simulink model "ASM_FOC_Implementation"  (R2020a)
settings: Solver=ode3  StartTime=0.0  StopTime=t_end  FixedStep=dt  RelTol=1e-3  EnableMultiTasking=on
values from neighbouring files (symbols this model uses):
  L_m = 0.326    [Experiment_4_Parameter.m]
  L_r = 0.340    (= 0.34)    [Experiment_4_Parameter.m]
  L_s = 0.340    (= 0.34)    [Experiment_4_Parameter.m]
  L_sigma_r = L_r - L_m    (= 0.014)    [Experiment_4_Parameter.m]
  L_sigma_s = L_s - L_m    (= 0.014)    [Experiment_4_Parameter.m]
  p = 1    [Experiment_4_Parameter.m]
  R_r = 2.9    [Experiment_4_Parameter.m]
  R_s = 2.3    [Experiment_4_Parameter.m]
  sigma = (L_s*L_r - L_m^2)/(L_s*L_r)    (= 0.0806574394464)    [Experiment_4_Parameter.m]
  T_c = 1/4000    (= 0.00025)    [Experiment_4_Parameter.m]
  Theta_M = 0.0022    [Experiment_4_Parameter.m]
  U_dc = 560    [Experiment_4_Parameter.m]
settings Model: Creator=julien  LastModifiedBy=ge29wel
settings DataIOCC: LimitDataPoints=on  SaveFormat=Array  ReturnWorkspaceOutputs=off
settings OptimizationCC: ExpressionDepthLimit=2147483647  LifeSpan=inf
settings DebuggingCC: UnderspecifiedInitializationDetection=Classic  MergeDetectMultiDrivingBlocksExec=none  SolverPrmCheckMsg=warning  MultiTaskRateTransMsg=warning  StateNameClashWarn=warning  SFUnexpectedBacktrackingDiag=warning  SFNoUnconditionalDefaultTransitionDiag=warning  SFExecutionAtInitializationDiag=none  ArithmeticOperatorsInVariantConditions=warning
settings HardwareCC: ProdBitPerPointer=32  ProdBitPerSizeT=32  ProdBitPerPtrDiffT=32  ProdLargestAtomicFloat=None  ProdIntDivRoundTo=Undefined  ProdEndianess=Unspecified  ProdWordSize=32  ProdHWDeviceType=32-bit Generic
settings ModelReferenceCC: PropagateSignalLabelsOutOfModel=off
settings SFSimCC: SimUseLocalCustomCode=off  CustomCodeUndefinedFunction=UseInterfaceOnly
settings RTWCC: RTWUseLocalCustomCode=off
settings CodeAppCC: StateflowObjectComments=on
settings GRTTargetCC: TargetLangStandard=C89/C90 (ANSI)
settings ConfigComp: CovMetricSettings=dw  CovHtmlReporting=on  CovSaveCumulativeToWorkspaceVar=on  CovSaveSingleToWorkspaceVar=on  CovExternalEMLEnable=off  CovSFcnEnable=off
settings ConfigurationSet: Description=SimMechanics 2G

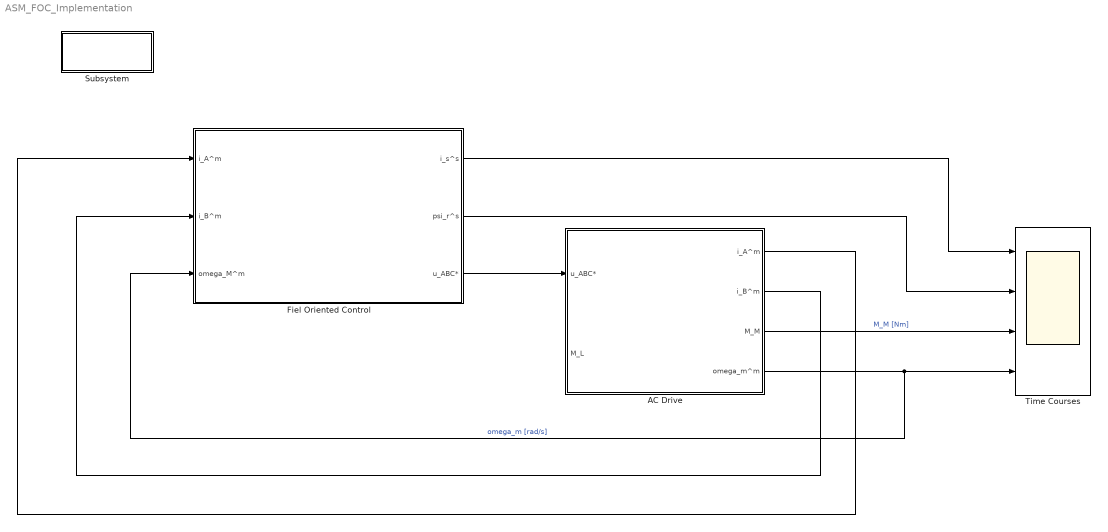
== system ASM_FOC_Implementation ==
  AC Drive : Subsystem
  Fiel Oriented Control : Subsystem
  Subsystem : Subsystem
      settings: OpenFcn=Experiment_4_Parameter
      mask Display: disp('Initialize\n (doppelklicken)')
  Time Courses : Scope  NumInputPorts=4
  wires:
  AC Drive/4(omega_m^m) -> Time Courses/4, Fiel Oriented Control/3(omega_M^m)  "omega_m [rad/s]"
  AC Drive/3(M_M) -> Time Courses/3  "M_M [Nm]"
  AC Drive/1(i_A^m) -> Fiel Oriented Control/1(i_A^m)
  AC Drive/2(i_B^m) -> Fiel Oriented Control/2(i_B^m)
  Fiel Oriented Control/1(i_s^s) -> Time Courses/1
  Fiel Oriented Control/3(u_ABC*) -> AC Drive/1(u_ABC*)
  Fiel Oriented Control/2(psi_r^s) -> Time Courses/2

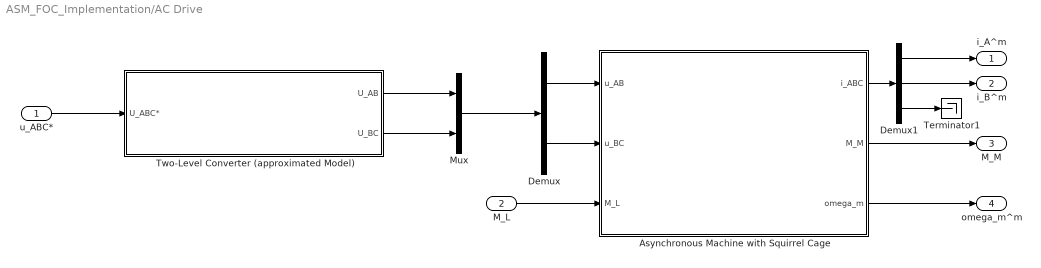
== system ASM_FOC_Implementation/AC Drive ==
  u_ABC* : Inport
  M_L : Inport  Port=2
  Asynchronous Machine with Squirrel Cage : Subsystem
  Demux : Demux  Outputs=2
  Demux1 : Demux  Outputs=3
  Mux : Mux  Inputs=2
  Terminator1 : Terminator
  Two-Level Converter (approximated Model) : Subsystem
  i_A^m : Outport
  i_B^m : Outport  Port=2
  M_M : Outport  Port=3
  omega_m^m : Outport  Port=4
  wires:
  Asynchronous Machine with Squirrel Cage/2(M_M) -> M_M/1
  M_L/1 -> Asynchronous Machine with Squirrel Cage/3(M_L)
  u_ABC*/1 -> Two-Level Converter (approximated Model)/1(U_ABC*)
  Demux/1 -> Asynchronous Machine with Squirrel Cage/1(u_AB)
  Demux/2 -> Asynchronous Machine with Squirrel Cage/2(u_BC)
  Two-Level Converter (approximated Model)/1(U_AB) -> Mux/1
  Two-Level Converter (approximated Model)/2(U_BC) -> Mux/2
  Mux/1 -> Demux/1
  Asynchronous Machine with Squirrel Cage/1(i_ABC) -> Demux1/1
  Demux1/3 -> Terminator1/1
  Asynchronous Machine with Squirrel Cage/3(omega_m) -> omega_m^m/1
  Demux1/1 -> i_A^m/1
  Demux1/2 -> i_B^m/1

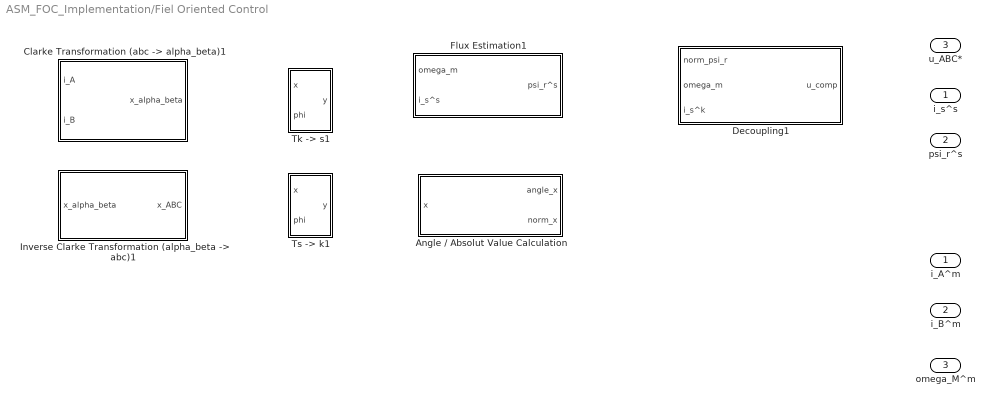
== system ASM_FOC_Implementation/Fiel Oriented Control ==
  i_A^m : Inport
  i_B^m : Inport  Port=2
  omega_M^m : Inport  Port=3
  "Angle / Absolut Value Calculation " : Subsystem
  "Clarke Transformation (abc -> alpha_beta)1" : Subsystem
  Decoupling1 : Subsystem
  Flux Estimation1 : Subsystem
  "Inverse Clarke Transformation (alpha_beta -> abc)1" : Subsystem
  "Tk -> s1" : Subsystem
  "Ts -> k1" : Subsystem
  i_s^s : Outport
  psi_r^s : Outport  Port=2
  u_ABC* : Outport  Port=3

== system ASM_FOC_Implementation/Subsystem ==

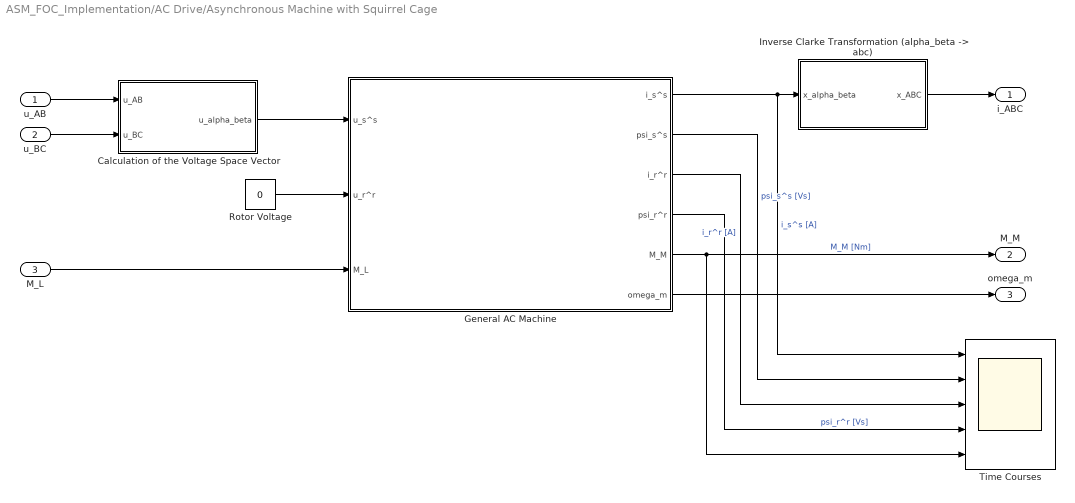
== system ASM_FOC_Implementation/AC Drive/Asynchronous Machine with Squirrel Cage ==
  u_AB : Inport
  u_BC : Inport  Port=2
  M_L : Inport  Port=3
  Calculation of the Voltage Space Vector : Subsystem
  General AC Machine : Subsystem
  "Inverse Clarke Transformation (alpha_beta -> abc)" : Subsystem
  Rotor Voltage : Constant  Value=0
  Time Courses : Scope  NumInputPorts=5
  i_ABC : Outport
  M_M : Outport  Port=2
  omega_m : Outport  Port=3
  wires:
  Rotor Voltage/1 -> General AC Machine/2(u_r^r)
  Calculation of the Voltage Space Vector/1(u_alpha_beta) -> General AC Machine/1(u_s^s)
  General AC Machine/1(i_s^s) -> Time Courses/1, "Inverse Clarke Transformation (alpha_beta -> abc)"/1(x_alpha_beta)  "i_s^s [A]"
  M_L/1 -> General AC Machine/3(M_L)
  General AC Machine/5(M_M) -> Time Courses/5, M_M/1  "M_M [Nm]"
  "Inverse Clarke Transformation (alpha_beta -> abc)"/1(x_ABC) -> i_ABC/1
  General AC Machine/6(omega_m) -> omega_m/1
  u_AB/1 -> Calculation of the Voltage Space Vector/1(u_AB)
  u_BC/1 -> Calculation of the Voltage Space Vector/2(u_BC)
  General AC Machine/2(psi_s^s) -> Time Courses/2  "psi_s^s [Vs]"
  General AC Machine/3(i_r^r) -> Time Courses/3  "i_r^r [A]"
  General AC Machine/4(psi_r^r) -> Time Courses/4  "psi_r^r [Vs]"

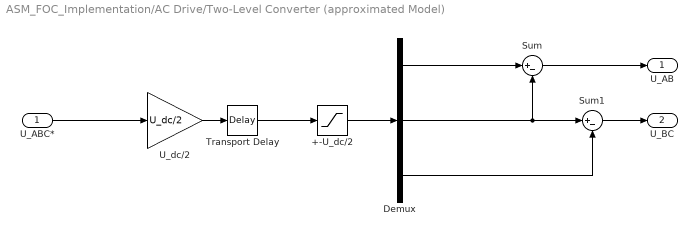
== system ASM_FOC_Implementation/AC Drive/Two-Level Converter (approximated Model) ==
  U_ABC* : Inport
  +-U_dc/2 : Saturate  UpperLimit=0.5*U_dc  LowerLimit=-0.5*U_dc
  Demux : Demux  Outputs=3
  Sum : Sum  Inputs=|+-
  Sum1 : Sum  Inputs=|+-
  Transport Delay : TransportDelay  DelayTime=T_c
  "U_dc/2 " : Gain  Gain=U_dc/2
  U_AB : Outport
  U_BC : Outport  Port=2
  wires:
  U_ABC*/1 -> "U_dc/2 "/1
  Sum1/1 -> U_BC/1
  Sum/1 -> U_AB/1
  "U_dc/2 "/1 -> Transport Delay/1
  Demux/3 -> Sum1/2
  Demux/1 -> Sum/1
  Demux/2 -> Sum1/1, Sum/2
  Transport Delay/1 -> +-U_dc/2/1
  +-U_dc/2/1 -> Demux/1

== system ASM_FOC_Implementation/Fiel Oriented Control/Angle // Absolut Value Calculation  ==
  x : Inport
  Demux : Demux  Outputs=2
  Math Function : Math  Operator=square  SignedPower=on  SaturateOnIntegerOverflow=on
  Math Function1 : Math  Operator=square  SignedPower=on  SaturateOnIntegerOverflow=on
  Sqrt : Sqrt  SaturateOnIntegerOverflow=on
  Sum1 : Sum  Inputs=+|+
  Trigonometric Function : Trigonometry  Operator=atan2
  angle_x : Outport
  norm_x : Outport  Port=2
  wires:
  Demux/2 -> Math Function1/1, Trigonometric Function/1
  Demux/1 -> Math Function/1, Trigonometric Function/2
  Trigonometric Function/1 -> angle_x/1
  Math Function1/1 -> Sum1/1
  Sum1/1 -> Sqrt/1
  Math Function/1 -> Sum1/2
  Sqrt/1 -> norm_x/1
  x/1 -> Demux/1

== system ASM_FOC_Implementation/Fiel Oriented Control/Clarke Transformation (abc -> alpha_beta)1 ==
  i_A : Inport
  i_B : Inport  Port=2
  2 : Gain  Gain=2
  Mux2 : Mux  Inputs=2
  Sum : Sum  Inputs=++|
  sqrt(3)/3 : Gain  Gain=sqrt(3)/3
  x_alpha_beta : Outport
  wires:
  i_A/1 -> Sum/1, Mux2/1
  i_B/1 -> 2/1
  Sum/1 -> sqrt(3)/3/1
  sqrt(3)/3/1 -> Mux2/2
  Mux2/1 -> x_alpha_beta/1
  2/1 -> Sum/2

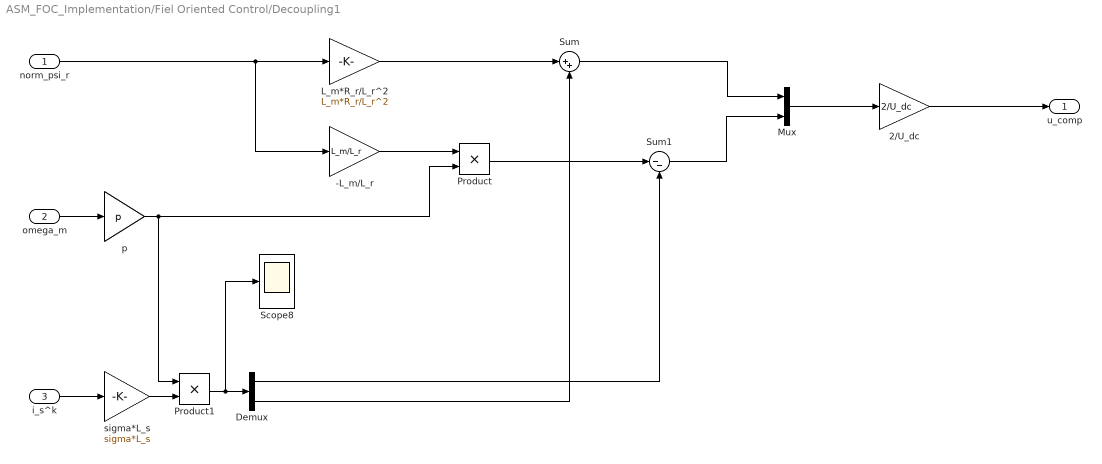
== system ASM_FOC_Implementation/Fiel Oriented Control/Decoupling1 ==
  norm_psi_r : Inport
  omega_m : Inport  Port=2
  i_s^k : Inport  Port=3
  -L_m/L_r : Gain  Gain=L_m/L_r
  2/U_dc : Gain  Gain=2/U_dc
  Demux : Demux  Outputs=2
  L_m*R_r/L_r^2 : Gain  Gain=L_m*R_r/L_r^2
  Mux : Mux  Inputs=2
  Product : Product  RndMeth=Zero
  Product1 : Product  RndMeth=Zero
  Scope8 : Scope
  Sum : Sum  Inputs=|++
  Sum1 : Sum  Inputs=|--
  p : Gain  Gain=p
  sigma*L_s : Gain  Gain=sigma*L_s
  u_comp : Outport
  wires:
  omega_m/1 -> p/1
  norm_psi_r/1 -> -L_m/L_r/1, L_m*R_r/L_r^2/1
  i_s^k/1 -> sigma*L_s/1
  -L_m/L_r/1 -> Product/1
  p/1 -> Product1/1, Product/2
  sigma*L_s/1 -> Product1/2
  Product1/1 -> Scope8/1, Demux/1
  L_m*R_r/L_r^2/1 -> Sum/1
  Demux/2 -> Sum/2
  Product/1 -> Sum1/1
  Demux/1 -> Sum1/2
  Mux/1 -> 2/U_dc/1
  Sum/1 -> Mux/1
  Sum1/1 -> Mux/2
  2/U_dc/1 -> u_comp/1

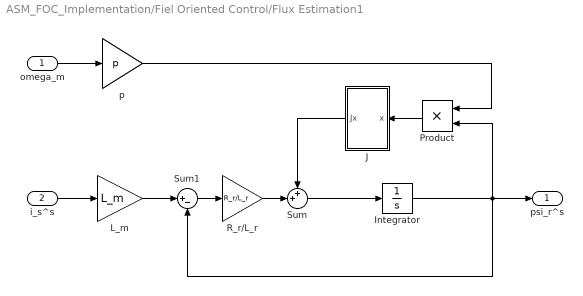
== system ASM_FOC_Implementation/Fiel Oriented Control/Flux Estimation1 ==
  omega_m : Inport
  i_s^s : Inport  Port=2
  Integrator : Integrator
  J : Subsystem
  L_m : Gain  Gain=L_m
  Product : Product  RndMeth=Zero
  R_r/L_r : Gain  Gain=R_r/L_r
  Sum : Sum  Inputs=++|
  Sum1 : Sum  Inputs=|+-
  p : Gain  Gain=p
  psi_r^s : Outport
  wires:
  L_m/1 -> Sum1/1
  Product/1 -> J/1(x)
  J/1(Jx) -> Sum/1
  i_s^s/1 -> L_m/1
  Sum/1 -> Integrator/1
  R_r/L_r/1 -> Sum/2
  Sum1/1 -> R_r/L_r/1
  Integrator/1 -> psi_r^s/1, Sum1/2, Product/2
  omega_m/1 -> p/1
  p/1 -> Product/1

== system ASM_FOC_Implementation/Fiel Oriented Control/Inverse Clarke Transformation (alpha_beta -> abc)1 ==
  x_alpha_beta : Inport
  "1/2 " : Gain  Gain=1/2
  Demux : Demux  Outputs=2
  Mux2 : Mux  Inputs=3
  Sum : Sum  Inputs=|-+
  Sum1 : Sum  Inputs=|--
  sqrt(3)/2 : Gain  Gain=sqrt(3)/2
  x_ABC : Outport
  wires:
  x_alpha_beta/1 -> Demux/1
  Demux/1 -> Mux2/1, "1/2 "/1
  Mux2/1 -> x_ABC/1
  Demux/2 -> sqrt(3)/2/1
  "1/2 "/1 -> Sum/1, Sum1/1
  sqrt(3)/2/1 -> Sum/2, Sum1/2
  Sum/1 -> Mux2/2
  Sum1/1 -> Mux2/3

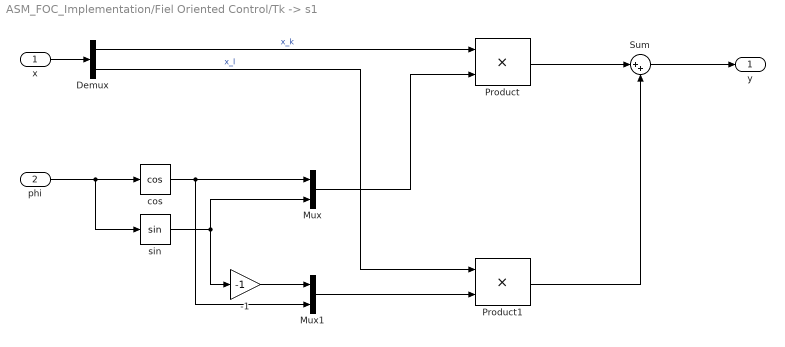
== system ASM_FOC_Implementation/Fiel Oriented Control/Tk -> s1 ==
  x : Inport
  phi : Inport  Port=2
  -1 : Gain  Gain=-1
  Demux : Demux  Outputs=2
  Mux : Mux  Inputs=2
  Mux1 : Mux  Inputs=2
  Product : Product  RndMeth=Zero
  Product1 : Product  RndMeth=Zero
  Sum : Sum  Inputs=|++
  cos : Trigonometry  Operator=cos
  sin : Trigonometry
  y : Outport
  wires:
  x/1 -> Demux/1
  phi/1 -> cos/1, sin/1
  cos/1 -> Mux/1, Mux1/2
  sin/1 -> Mux/2, -1/1
  Mux/1 -> Product/2
  -1/1 -> Mux1/1
  Mux1/1 -> Product1/2
  Demux/2 -> Product1/1  "x_l"
  Product/1 -> Sum/1
  Product1/1 -> Sum/2
  Sum/1 -> y/1
  Demux/1 -> Product/1  "x_k"

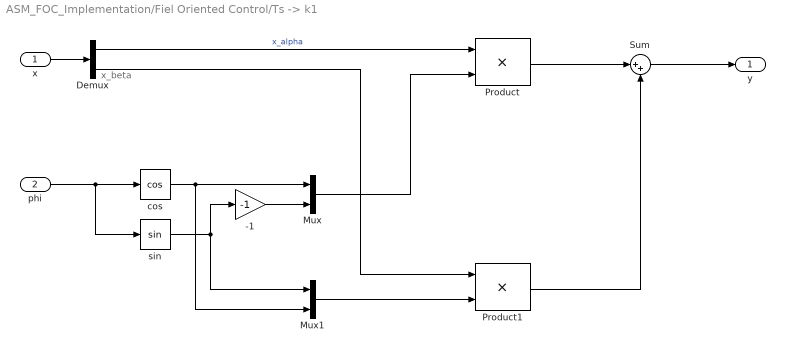
== system ASM_FOC_Implementation/Fiel Oriented Control/Ts -> k1 ==
  note: x_beta
  x : Inport
  phi : Inport  Port=2
  -1 : Gain  Gain=-1
  Demux : Demux  Outputs=2
  Mux : Mux  Inputs=2
  Mux1 : Mux  Inputs=2
  Product : Product  RndMeth=Zero
  Product1 : Product  RndMeth=Zero
  Sum : Sum  Inputs=|++
  cos : Trigonometry  Operator=cos
  sin : Trigonometry
  y : Outport
  wires:
  x/1 -> Demux/1
  phi/1 -> cos/1, sin/1
  Demux/1 -> Product/1  "x_alpha"
  cos/1 -> Mux/1, Mux1/2
  sin/1 -> -1/1, Mux1/1
  Mux/1 -> Product/2
  Mux1/1 -> Product1/2
  Demux/2 -> Product1/1
  Product/1 -> Sum/1
  Product1/1 -> Sum/2
  -1/1 -> Mux/2
  Sum/1 -> y/1

== system ASM_FOC_Implementation/AC Drive/Asynchronous Machine with Squirrel Cage/Calculation of the Voltage Space Vector ==
  u_AB : Inport
  u_BC : Inport  Port=2
  1/3 : Gain  Gain=1/3
  2/3 : Gain  Gain=2/3
  Mux2 : Mux  Inputs=2
  Sum : Sum  Inputs=|++
  sqrt(3)/3 : Gain  Gain=sqrt(3)/3
  u_alpha_beta : Outport
  wires:
  Mux2/1 -> u_alpha_beta/1
  u_AB/1 -> 2/3/1
  u_BC/1 -> sqrt(3)/3/1, 1/3/1
  2/3/1 -> Sum/1
  1/3/1 -> Sum/2
  Sum/1 -> Mux2/1
  sqrt(3)/3/1 -> Mux2/2

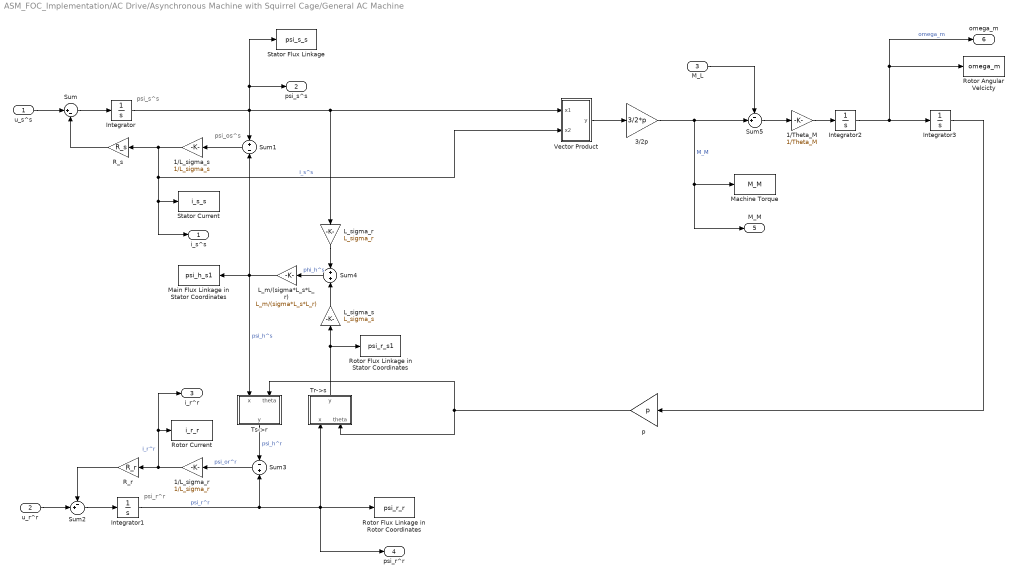
== system ASM_FOC_Implementation/AC Drive/Asynchronous Machine with Squirrel Cage/General AC Machine ==
  note: psi_s^s
  note: psi_r^r
  note: psi_os^s
  u_s^s : Inport
  u_r^r : Inport  Port=2
  M_L : Inport  Port=3
  1/L_sigma_r : Gain  Gain=1/L_sigma_r
  1/L_sigma_s : Gain  Gain=1/L_sigma_s
  1/Theta_M : Gain  Gain=1/Theta_M
  3/2p : Gain  Gain=3/2*p
  Integrator{,1..3} (4 alike) : Integrator
  L_m/(sigma*L_s*L_r) : Gain  Gain=L_m/(sigma*L_s*L_r)
  L_sigma_r : Gain  Gain=L_sigma_r
  L_sigma_s : Gain  Gain=L_sigma_s
  Machine Torque : ToWorkspace  VariableName=M_M  SaveFormat=Timeseries  SampleTime=-1
  "Main Flux Linkage in Stator Coordinates " : ToWorkspace  VariableName=psi_h_s1  SaveFormat=Timeseries  SampleTime=-1
  R_r : Gain  Gain=R_r
  R_s : Gain  Gain=R_s
  Rotor Angular Velcicty : ToWorkspace  VariableName=omega_m  SaveFormat=Timeseries  SampleTime=-1
  Rotor Current : ToWorkspace  VariableName=i_r_r  SaveFormat=Timeseries  SampleTime=-1
  Rotor Flux Linkage in Rotor Coordinates : ToWorkspace  VariableName=psi_r_r  SaveFormat=Timeseries  SampleTime=-1
  "Rotor Flux Linkage in Stator Coordinates " : ToWorkspace  VariableName=psi_r_s1  SaveFormat=Timeseries  SampleTime=-1
  Stator Current : ToWorkspace  VariableName=i_s_s  SaveFormat=Timeseries  SampleTime=-1
  Stator Flux Linkage : ToWorkspace  VariableName=psi_s_s  SaveFormat=Timeseries  SampleTime=-1
  Sum : Sum  Inputs=|+-
  Sum1 : Sum  Inputs=+|-
  Sum2 : Sum  Inputs=-+|
  Sum3 : Sum  Inputs=-|+
  Sum4 : Sum  Inputs=+|+
  Sum5 : Sum  Inputs=-+|
  Tr->s : Subsystem
  Ts->r : Subsystem
  Vector Product : Subsystem
  p : Gain  Gain=p
  i_s^s : Outport
  psi_s^s : Outport  Port=2
  i_r^r : Outport  Port=3
  psi_r^r : Outport  Port=4
  M_M : Outport  Port=5
  omega_m : Outport  Port=6
  wires:
  u_s^s/1 -> Sum/1
  R_s/1 -> Sum/2
  Sum/1 -> Integrator/1
  1/L_sigma_s/1 -> R_s/1, Stator Current/1, i_s^s/1, Vector Product/2(x2)  "i_s^s"
  Integrator/1 -> psi_s^s/1, Stator Flux Linkage/1, Sum1/1, L_sigma_r/1, Vector Product/1(x1)
  Sum1/1 -> 1/L_sigma_s/1
  u_r^r/1 -> Sum2/2
  Sum2/1 -> Integrator1/1
  R_r/1 -> Sum2/1
  1/L_sigma_r/1 -> R_r/1, Rotor Current/1, i_r^r/1  "i_r^r"
  Integrator1/1 -> Sum3/2, psi_r^r/1, Tr->s/1(x), Rotor Flux Linkage in Rotor Coordinates/1  "psi_r^r"
  Sum3/1 -> 1/L_sigma_r/1  "psi_or^r"
  Tr->s/1(y) -> "Rotor Flux Linkage in Stator Coordinates "/1, L_sigma_s/1
  L_sigma_r/1 -> Sum4/1
  L_sigma_s/1 -> Sum4/2
  Vector Product/1(y) -> 3/2p/1
  3/2p/1 -> Machine Torque/1, M_M/1, Sum5/2  "M_M"
  M_L/1 -> Sum5/1
  Sum5/1 -> 1/Theta_M/1
  1/Theta_M/1 -> Integrator2/1
  Integrator2/1 -> Integrator3/1, Rotor Angular Velcicty/1, omega_m/1  "omega_m"
  Integrator3/1 -> p/1
  Ts->r/1(y) -> Sum3/1  "psi_h^r"
  L_m/(sigma*L_s*L_r)/1 -> "Main Flux Linkage in Stator Coordinates "/1, Sum1/2, Ts->r/1(x)  "psi_h^s"
  p/1 -> Ts->r/2(theta), Tr->s/2(theta)
  Sum4/1 -> L_m/(sigma*L_s*L_r)/1  "phi_h^s"

== system ASM_FOC_Implementation/AC Drive/Asynchronous Machine with Squirrel Cage/Inverse Clarke Transformation (alpha_beta -> abc) ==
  x_alpha_beta : Inport
  "1/2 " : Gain  Gain=1/2
  Demux : Demux  Outputs=2
  Mux2 : Mux  Inputs=3
  Sum : Sum  Inputs=|-+
  Sum1 : Sum  Inputs=|--
  sqrt(3)/2 : Gain  Gain=sqrt(3)/2
  x_ABC : Outport
  wires:
  x_alpha_beta/1 -> Demux/1
  Demux/1 -> Mux2/1, "1/2 "/1
  Mux2/1 -> x_ABC/1
  Demux/2 -> sqrt(3)/2/1
  "1/2 "/1 -> Sum/1, Sum1/1
  sqrt(3)/2/1 -> Sum/2, Sum1/2
  Sum/1 -> Mux2/2
  Sum1/1 -> Mux2/3

== system ASM_FOC_Implementation/Fiel Oriented Control/Flux Estimation1/J ==
  note: x_beta
  x : Inport
  -1 : Gain  Gain=-1
  Demux : Demux  Outputs=2
  Mux : Mux  Inputs=2
  Jx : Outport
  wires:
  x/1 -> Demux/1
  Demux/1 -> Mux/2  "x_alpha"
  Demux/2 -> -1/1
  Mux/1 -> Jx/1
  -1/1 -> Mux/1

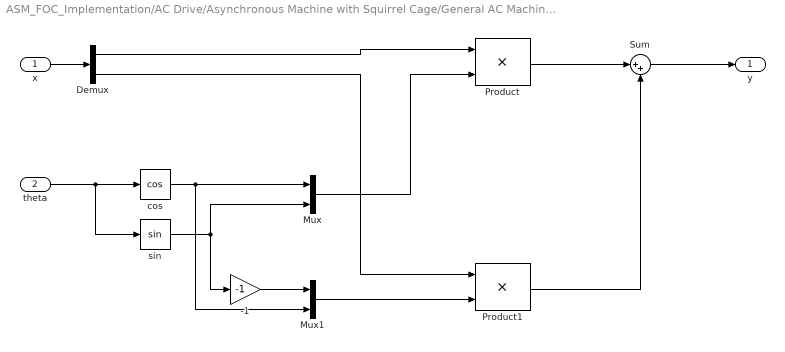
== system ASM_FOC_Implementation/AC Drive/Asynchronous Machine with Squirrel Cage/General AC Machine/Tr->s ==
  x : Inport
  theta : Inport  Port=2
  -1 : Gain  Gain=-1
  Demux : Demux  Outputs=2
  Mux : Mux  Inputs=2
  Mux1 : Mux  Inputs=2
  Product : Product  RndMeth=Zero
  Product1 : Product  RndMeth=Zero
  Sum : Sum  Inputs=|++
  cos : Trigonometry  Operator=cos
  sin : Trigonometry
  y : Outport
  wires:
  x/1 -> Demux/1
  theta/1 -> cos/1, sin/1
  cos/1 -> Mux/1, Mux1/2
  sin/1 -> Mux/2, -1/1
  Mux/1 -> Product/2
  -1/1 -> Mux1/1
  Mux1/1 -> Product1/2
  Demux/2 -> Product1/1
  Product/1 -> Sum/1
  Product1/1 -> Sum/2
  Sum/1 -> y/1
  Demux/1 -> Product/1

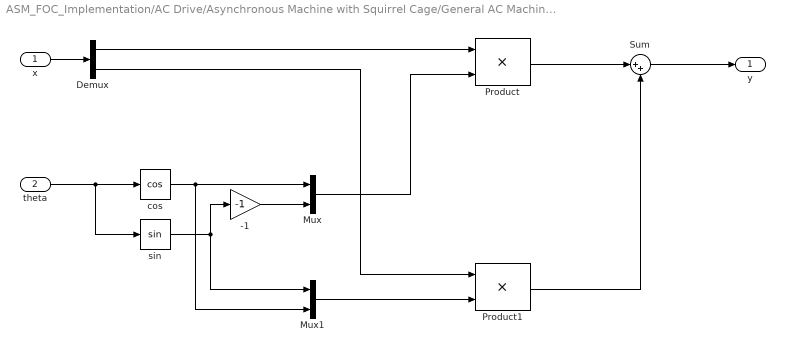
== system ASM_FOC_Implementation/AC Drive/Asynchronous Machine with Squirrel Cage/General AC Machine/Ts->r ==
  x : Inport
  theta : Inport  Port=2
  -1 : Gain  Gain=-1
  Demux : Demux  Outputs=2
  Mux : Mux  Inputs=2
  Mux1 : Mux  Inputs=2
  Product : Product  RndMeth=Zero
  Product1 : Product  RndMeth=Zero
  Sum : Sum  Inputs=|++
  cos : Trigonometry  Operator=cos
  sin : Trigonometry
  y : Outport
  wires:
  x/1 -> Demux/1
  theta/1 -> cos/1, sin/1
  Demux/1 -> Product/1
  cos/1 -> Mux/1, Mux1/2
  sin/1 -> -1/1, Mux1/1
  Mux/1 -> Product/2
  Mux1/1 -> Product1/2
  Demux/2 -> Product1/1
  Product/1 -> Sum/1
  Product1/1 -> Sum/2
  -1/1 -> Mux/2
  Sum/1 -> y/1

== system ASM_FOC_Implementation/AC Drive/Asynchronous Machine with Squirrel Cage/General AC Machine/Vector Product ==
  x1 : Inport
  x2 : Inport  Port=2
  Demux : Demux  Outputs=2
  Demux1 : Demux  Outputs=2
  Product : Product  RndMeth=Zero
  Product1 : Product  RndMeth=Zero
  Sum : Sum  Inputs=|+-
  y : Outport
  wires:
  Sum/1 -> y/1
  Product1/1 -> Sum/2
  Product/1 -> Sum/1
  Demux1/1 -> Product1/2
  Demux/2 -> Product1/1
  Demux1/2 -> Product/2
  Demux/1 -> Product/1
  x2/1 -> Demux1/1
  x1/1 -> Demux/1
